simulink model "modelo"  (R2015a)
settings: Solver=ode1  SolverMode=SingleTasking  StartTime=0.0  StopTime=10  FixedStep=0.01  RelTol=1e-3
values from neighbouring files (symbols this model uses):
  K = 54.93    [exp7.m]
  KNL = 59.85    [exp7.m]
  Kp = 1.633    [CtrlPos_P_Kc05.mat]    (also in CtrlPos_P_Kc10.mat; CtrlPos_P_Kc15.mat; exp7.m = 1.59)
  Kpi = 0.661 / tr(i)    [exp7.m]
  KtL = KKt / K    (= 0.0169)    [exp7.m]
  KtNL = KKt / KNL    (= 0.015510726817)    [exp7.m]
  phi = 1.2    [exp7.m]
  T = 0.28    [exp7.m]
  Ti = T    (= 0.28)    [exp7.m]
  U = Kp * pi / 2    (= 2.4975661596)    [exp7.m]
settings Model: CovExternalEMLEnable=on  Creator=rpm  LastModifiedBy=natanael
settings DataIOCC: LimitDataPoints=off  SignalLoggingSaveFormat=ModelDataLogs  SaveOutput=off  SignalLogging=off  DSMLogging=off  SaveTime=off  TimeSaveName=t
settings OptimizationCC: ExpressionDepthLimit=2147483647  InitFltsAndDblsToZero=on
settings DebuggingCC: UnderspecifiedInitializationDetection=Classic  MergeDetectMultiDrivingBlocksExec=none  FcnCallInpInsideContextMsg=EnableAllAsWarning  StateNameClashWarn=warning
settings GRTTargetCC: CombineOutputUpdateFcns=off  GRTInterface=on

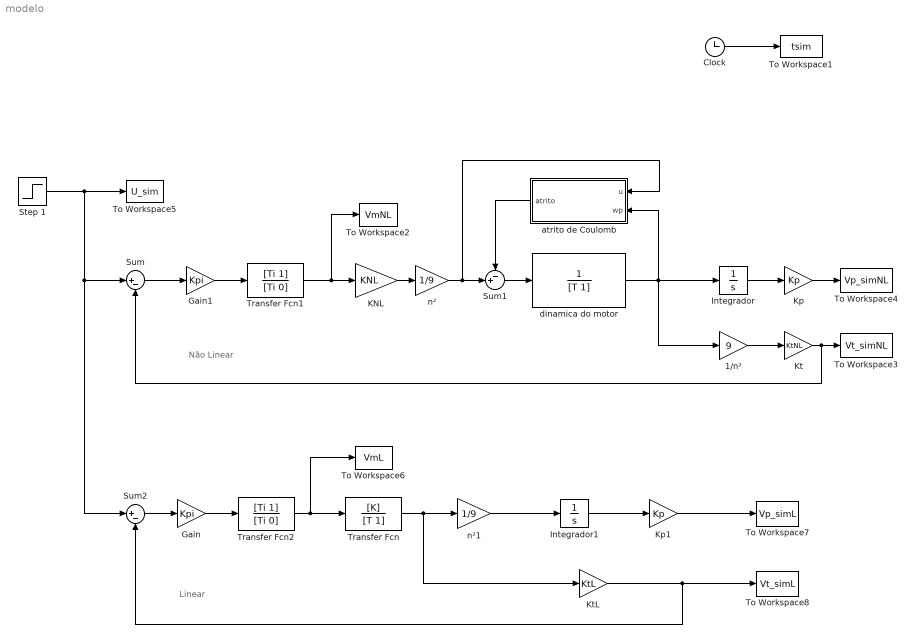
== system modelo ==
  note: Não Linear
  note: Linear
  1/n² : Gain  Gain=9
  Clock : Clock
  Gain : Gain  Gain=Kpi
  Gain1 : Gain  Gain=Kpi
  Integrador : Integrator
  Integrador1 : Integrator
  KNL : Gain  Gain=KNL
  Kp : Gain  Gain=Kp
  Kp1 : Gain  Gain=Kp
  Kt : Gain  Gain=KtNL
  KtL : Gain  Gain=KtL
  Step 1 : Step  After=U  SampleTime=0
  Sum : Sum  Inputs=|+-
  Sum1 : Sum  Inputs=-+|
  Sum2 : Sum  Inputs=|+-
  To Workspace1 : ToWorkspace  VariableName=tsim  SampleTime=-1
  To Workspace2 : ToWorkspace  VariableName=VmNL  SampleTime=-1
  To Workspace3 : ToWorkspace  VariableName=Vt_simNL  SampleTime=-1
  To Workspace4 : ToWorkspace  VariableName=Vp_simNL  SampleTime=-1
  To Workspace5 : ToWorkspace  VariableName=U_sim  SampleTime=-1
  To Workspace6 : ToWorkspace  VariableName=VmL  SampleTime=-1
  To Workspace7 : ToWorkspace  VariableName=Vp_simL  SampleTime=-1
  To Workspace8 : ToWorkspace  VariableName=Vt_simL  SampleTime=-1
  Transfer Fcn : TransferFcn  Numerator=[K]  Denominator=[T 1]
  Transfer Fcn1 : TransferFcn  Numerator=[Ti 1]  Denominator=[Ti 0]
  Transfer Fcn2 : TransferFcn  Numerator=[Ti 1]  Denominator=[Ti 0]
  atrito de Coulomb : Subsystem  mask{phi=phi}
      mask Display: fprintf('phi = %3.1f', phi)
  dinamica do motor : TransferFcn  Denominator=[T 1]
  n² : Gain  Gain=1/9
  n²1 : Gain  Gain=1/9
  wires:
  dinamica do motor/1 -> 1/n²/1, Integrador/1, atrito de Coulomb/2(wp)
  Integrador/1 -> Kp/1
  Kt/1 -> Sum/2, To Workspace3/1
  Kp/1 -> To Workspace4/1
  KNL/1 -> n²/1
  n²/1 -> atrito de Coulomb/1(u), Sum1/2
  atrito de Coulomb/1(atrito) -> Sum1/1
  Sum1/1 -> dinamica do motor/1
  1/n²/1 -> Kt/1
  Transfer Fcn1/1 -> To Workspace2/1, KNL/1
  Step 1/1 -> To Workspace5/1, Sum2/1, Sum/1
  Clock/1 -> To Workspace1/1
  Transfer Fcn2/1 -> To Workspace6/1, Transfer Fcn/1
  Transfer Fcn/1 -> KtL/1, n²1/1
  n²1/1 -> Integrador1/1
  Integrador1/1 -> Kp1/1
  Kp1/1 -> To Workspace7/1
  KtL/1 -> To Workspace8/1, Sum2/2
  Sum2/1 -> Gain/1
  Gain/1 -> Transfer Fcn2/1
  Sum/1 -> Gain1/1
  Gain1/1 -> Transfer Fcn1/1

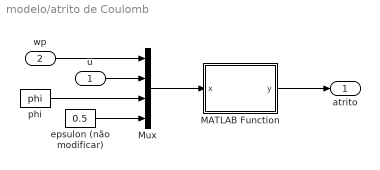
== system modelo/atrito de Coulomb ==
  u : Inport
  wp : Inport  Port=2
  MATLAB Function : MATLAB Function  TreatAsAtomicUnit=on
  Mux : Mux
  epsulon (não modificar) : Constant  Value=0.5
  phi : Constant  Value=phi
  atrito : Outport
  wires:
  u/1 -> Mux/2
  phi/1 -> Mux/3
  MATLAB Function/1(y) -> atrito/1
  wp/1 -> Mux/1
  epsulon (não modificar)/1 -> Mux/4
  Mux/1 -> MATLAB Function/1(x)

== matlab function modelo/atrito de Coulomb/MATLAB Function ==
  data: x input size=4; y output size=1
function y = nl_coulomb(x)
% Atrito de Coulomb
% Para uso de nl_template.mdl

wp  = x(1); 
u   = x(2); 
phi = x(3); 
epsulon = x(4);

y = 0;

if wp > epsulon
    y = phi;
elseif wp < -epsulon
    y = -phi;
elseif wp >= 0
    y = min(phi,abs(u));
elseif wp < 0
    y = max(-phi,-abs(u));
end
